simulink model "GFLIB_ControllerPIDpAW_BAM"  (Simulink 8.3)
settings: Solver=ode45  StartTime=0.0  StopTime=10.0  RelTol=1e-3
undefined symbols (not defined in the file): f16DerivGain, f16FiltCoef, f16IntegGain, f16PropGain, s16DerivGainShift, s16IntegGainShift, s16PropGainShift
settings Model: Creator=nxf41029  LastModifiedBy=nxf41029
settings DataIOCC: SignalLoggingSaveFormat=Dataset
settings DebuggingCC: UnderspecifiedInitializationDetection=Simplified  StateNameClashWarn=none
settings GRTTargetCC: CombineOutputUpdateFcns=on  GRTInterface=off

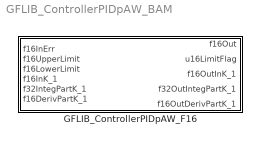
== system GFLIB_ControllerPIDpAW_BAM ==
  GFLIB_ControllerPIDpAW_F16 : Subsystem  mask(GFLIB_ControllerPIDpAW_F16){f16PropGain=f16PropGain, s16PropGainShift=s16PropGainShift, f16IntegGain=f16IntegGain, s16IntegGainShift=s16IntegGainShift, f16DerivGain=f16DerivGain, s16DerivGainShift=s16DerivGainShift, f16FiltCoef=f16FiltCoef}
      mask help: Bit accurate model of parallel form PID controller. All parameters as well as input and output are 16-bit integers except for s16xxxGainShift parameters which are 16-bit signed integers.
      mask init:
      | pos = get_param(gcb, 'Position');width = pos(3) - pos(1); height = pos(4) - pos(2);tX=width/2;tY=height*0.9;
      mask Display: color('black');port_label('input',1,'f16InErr');port_label('input',2,'f16UpperLimit');port_label('input',3,'f16LowerLimit');port_label('input',4,'f16InK_1');port_label('input',5,'f32IntegPartK_1');port_label('input',6,'f16DerivPartK_1');port_label('output',1,'f16Out');port_label('output',2,'u16LimitFlag');port_label('output',3,'f16OutInK_1');port_label('output',4,'f32OutIntegPartK_1');port_label('output',5,'f16OutDerivPartK_1');color('black');disp('GFLIB_ControllerPIDpAW_F16');color('blue');text(tX,tY, 'BAM', 'horizontalAlignment', 'center');

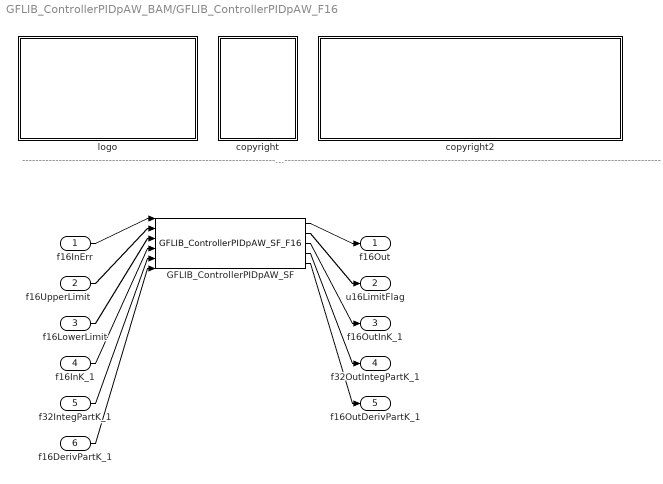
== system GFLIB_ControllerPIDpAW_BAM/GFLIB_ControllerPIDpAW_F16 ==
  note: ---------------------------------------------------------------------------------------------------------------------------------------------------------------------------------------------------
  f16InErr : Inport
  f16UpperLimit : Inport  Port=2
  f16LowerLimit : Inport  Port=3
  f16InK_1 : Inport  Port=4
  f32IntegPartK_1 : Inport  Port=5
  f16DerivPartK_1 : Inport  Port=6
  GFLIB_ControllerPIDpAW_SF : S-Function  FunctionName=GFLIB_ControllerPIDpAW_SF_F16  Parameters=f16PropGain,s16PropGainShift,f16IntegGain,s16IntegGainShift,f16DerivGain,s16DerivGainShift,f16FiltCoef  EnableBusSupport=off
  copyright : Subsystem
      mask Display: text(10,90,'FILE:');text(10,75,'DESRIPTION:');text(10,60,'COPYRIGHT:');text(10,45,'VERSION:');text(10,30,'DATE:')
  copyright2 : Subsystem
      mask Display: text(10,90,'GFLIB_ControllerPIDpAW_BAM_F16.mdl');text(10,75,'Parallel form of a standard PID controller with implemented anti-windup.');text(10,60,'NXP');text(10,45,'0.1');text(10,30,'21-Nov-2018');
  logo : Subsystem
      mask Display: image(imread('logo.jpg'))
  f16Out : Outport
  u16LimitFlag : Outport  Port=2
  f16OutInK_1 : Outport  Port=3
  f32OutIntegPartK_1 : Outport  Port=4
  f16OutDerivPartK_1 : Outport  Port=5
  wires:
  f16InErr/1 -> GFLIB_ControllerPIDpAW_SF/1
  f16UpperLimit/1 -> GFLIB_ControllerPIDpAW_SF/2
  f16LowerLimit/1 -> GFLIB_ControllerPIDpAW_SF/3
  f16InK_1/1 -> GFLIB_ControllerPIDpAW_SF/4
  f32IntegPartK_1/1 -> GFLIB_ControllerPIDpAW_SF/5
  f16DerivPartK_1/1 -> GFLIB_ControllerPIDpAW_SF/6
  GFLIB_ControllerPIDpAW_SF/1 -> f16Out/1
  GFLIB_ControllerPIDpAW_SF/2 -> u16LimitFlag/1
  GFLIB_ControllerPIDpAW_SF/3 -> f16OutInK_1/1
  GFLIB_ControllerPIDpAW_SF/4 -> f32OutIntegPartK_1/1
  GFLIB_ControllerPIDpAW_SF/5 -> f16OutDerivPartK_1/1

== system GFLIB_ControllerPIDpAW_BAM/GFLIB_ControllerPIDpAW_F16/copyright ==

== system GFLIB_ControllerPIDpAW_BAM/GFLIB_ControllerPIDpAW_F16/copyright2 ==

== system GFLIB_ControllerPIDpAW_BAM/GFLIB_ControllerPIDpAW_F16/logo ==
